simulink model "MILSIM"  (R2018b)
settings: Solver=FixedStepDiscrete  StartTime=0.0  StopTime=1000  FixedStep=0.002  RelTol=1e-3
undefined symbols (not defined in the file): alt, ax_cmd, ay_cmd, cmd_1, cmd_2, cmd_mask, command, DiscIntNeverNeededParam, FMS_Cmd, frame, lat, lon, mode, PilotMode, pitch, pitchspeed, psi_cmd, psi_rate_cmd, roll, rollspeed, serial, stick_pitch, stick_roll, stick_throttle, stick_yaw, timestamp, u_cmd, v_cmd, valid_items, VTOLMode, vx, vy, vz, x, x_cmd, xacc, y, y_cmd, yacc, yaw, yawspeed, z, z_cmd, zacc
libraries: hdlsllib x9, vrlib x2, instrumentlib x2, aerolibfltsims x2, aerolibutil x2, dspnetwork x2, simulink x1, aerolibanimutils x1
settings Model: Creator=jc  LastModifiedBy=spy
settings OptimizationCC: DefaultParameterBehavior=Inlined  DefaultUnderspecifiedDataType=single  EnhancedBackFolding=on  PassReuseOutputArgsAs=Individual arguments  OptimizeBlockOrder=speed  DifferentSizesBufferReuse=on  OptimizationCustomize=off
settings DebuggingCC: UnderspecifiedInitializationDetection=Classic  MergeDetectMultiDrivingBlocksExec=none  ParameterTunabilityLossMsg=error  UnitsInconsistencyMsg=none
settings HardwareCC: ProdBitPerPointer=32  ProdBitPerSizeT=32  ProdBitPerPtrDiffT=32  ProdLargestAtomicInteger=Long  ProdLargestAtomicFloat=Double  ProdWordSize=32  ProdHWDeviceType=ARM Compatible->ARM Cortex
settings ModelReferenceCC: UpdateModelReferenceTargets=IfOutOfDate  PropagateSignalLabelsOutOfModel=off
settings SFSimCC: MATLABDynamicMemAlloc=off
settings RTWCC: SystemTargetFile=ert.tlc  GenCodeOnly=on  TemplateMakefile=ert_default_tmf  GenerateReport=on  IncludeHyperlinkInReport=on  LaunchReport=on  GenerateTraceInfo=on  GenerateTraceReport=on  GenerateTraceReportSl=on  GenerateTraceReportSf=on  GenerateTraceReportEml=on
settings CodeAppCC: ForceParamTrailComments=on  IgnoreCustomStorageClasses=off  OperatorAnnotations=on  SimulinkDataObjDesc=on  SFDataObjDesc=on  InsertBlockDesc=on
settings ERTTargetCC: TargetLangStandard=C99 (ISO)  GenerateSampleERTMain=on  InlinedParameterPlacement=NonHierarchical  ERTCustomFileTemplate=example_file_process.tlc

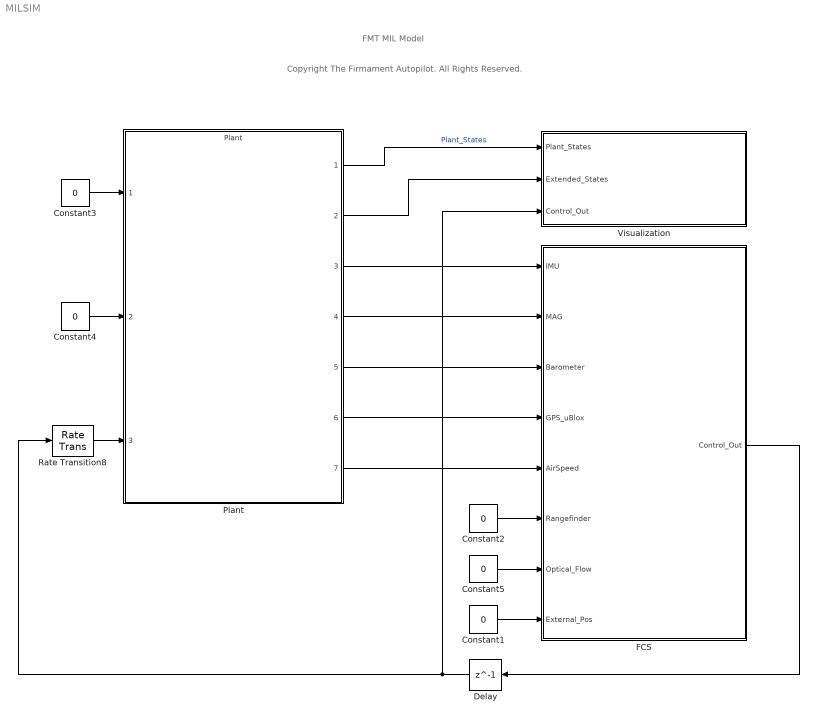
== system MILSIM ==
  note: FMT MIL Model
  note: Copyright The Firmament Autopilot. All Rights Reserved.
  Constant1 : Constant  Value=0  OutDataTypeStr=Bus: External_Pos_Bus
  Constant2 : Constant  Value=0  OutDataTypeStr=Bus: Rangefinder_Bus
  Constant3 : Constant  Value=0  OutDataTypeStr=Bus: Environment_Info_Bus
  Constant4 : Constant  Value=0  OutDataTypeStr=Bus: States_Init_Bus
  Constant5 : Constant  Value=0  OutDataTypeStr=Bus: Optical_Flow_Bus
  Delay : Delay  DelayLength=1
  FCS : Subsystem  TreatAsAtomicUnit=on
  Plant : ModelReference  ModelNameDialog=Plant.slx  ModelReferenceVersion=1.1206
  Rate Transition8 : RateTransition  OutPortSampleTime=PLANT_CONST.dt
  Visualization : Subsystem  TreatAsAtomicUnit=on
  wires:
  Plant/1 -> Visualization/1(Plant_States)  "Plant_States"
  Delay/1 -> Visualization/3(Control_Out), Rate Transition8/1
  Plant/2 -> Visualization/2(Extended_States)
  Plant/3 -> FCS/1(IMU)
  Plant/4 -> FCS/2(MAG)
  Plant/5 -> FCS/3(Barometer)
  FCS/1(Control_Out) -> Delay/1
  Constant2/1 -> FCS/6(Rangefinder)
  Constant5/1 -> FCS/7(Optical_Flow)
  Plant/7 -> FCS/5(AirSpeed)
  Constant1/1 -> FCS/8(External_Pos)
  Constant3/1 -> Plant/1
  Rate Transition8/1 -> Plant/3
  Constant4/1 -> Plant/2
  Plant/6 -> FCS/4(GPS_uBlox)

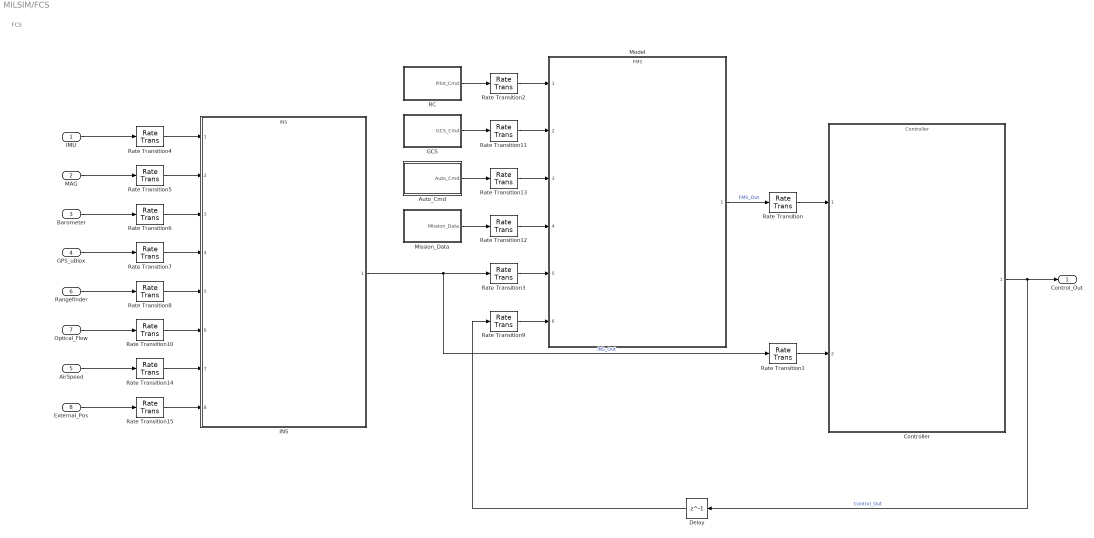
== system MILSIM/FCS ==
  note: FCS
  IMU : Inport
  MAG : Inport  Port=2
  Barometer : Inport  Port=3
  GPS_uBlox : Inport  Port=4
  AirSpeed : Inport  Port=5
  Rangefinder : Inport  Port=6
  Optical_Flow : Inport  Port=7
  External_Pos : Inport  Port=8
  Auto_Cmd : Subsystem
  Controller : ModelReference  ModelNameDialog=Controller.slx  ModelReferenceVersion=1.1001
  Delay : Delay  DelayLength=1
  GCS : Subsystem
  INS : ModelReference  ModelNameDialog=INS.slx  ModelReferenceVersion=1.4483
  Mission_Data : Subsystem
  Model : ModelReference  ModelNameDialog=FMS.slx  ModelReferenceVersion=1.2293
  RC : Subsystem  VariantControlMode=Label  Variant=on  VariantControl=Variant1  LabelModeActiveChoice=VIRTUAL_INPUT
  Rate Transition : RateTransition  OutPortSampleTime=CONTROL_CONST.dt
  Rate Transition1 : RateTransition  OutPortSampleTime=CONTROL_CONST.dt
  Rate Transition{4..8,10,14..15} (8 alike) : RateTransition  OutPortSampleTime=INS_CONST.dt
  Rate Transition{2..3,9,11..13} (6 alike) : RateTransition  OutPortSampleTime=FMS_CONST.dt
  Control_Out : Outport
  wires:
  INS/1 -> Rate Transition3/1, Rate Transition1/1  "INS_Out"
  Rate Transition2/1 -> Model/1
  Rate Transition4/1 -> INS/1
  Rate Transition/1 -> Controller/1
  Rate Transition1/1 -> Controller/2
  RC/1(" Pilot_Cmd") -> Rate Transition2/1
  Rangefinder/1 -> Rate Transition8/1
  Model/1 -> Rate Transition/1  "FMS_Out"
  Barometer/1 -> Rate Transition6/1
  Rate Transition3/1 -> Model/5
  MAG/1 -> Rate Transition5/1
  Rate Transition9/1 -> Model/6
  Controller/1 -> Delay/1, Control_Out/1  "Control_Out"
  IMU/1 -> Rate Transition4/1
  Delay/1 -> Rate Transition9/1
  Optical_Flow/1 -> Rate Transition10/1
  Rate Transition5/1 -> INS/2
  Rate Transition6/1 -> INS/3
  Rate Transition7/1 -> INS/4
  Rate Transition8/1 -> INS/5
  Rate Transition10/1 -> INS/6
  GPS_uBlox/1 -> Rate Transition7/1
  Rate Transition13/1 -> Model/3
  GCS/1(GCS_Cmd) -> Rate Transition11/1
  Rate Transition11/1 -> Model/2
  Mission_Data/1(Mission_Data) -> Rate Transition12/1
  Rate Transition12/1 -> Model/4
  Rate Transition14/1 -> INS/7
  Auto_Cmd/1(Auto_Cmd) -> Rate Transition13/1
  AirSpeed/1 -> Rate Transition14/1
  External_Pos/1 -> Rate Transition15/1
  Rate Transition15/1 -> INS/8

== system MILSIM/Visualization ==
  Plant_States : Inport
  Extended_States : Inport  Port=2
  Control_Out : Inport  Port=3
  3D_Visualization : Subsystem  VariantControlMode=Label  Variant=on  LabelModeActiveChoice=UE4
  Simulation Pace : aerolibanimutils/Simulation Pace  SimulationPace=1  SleepMode=Auto  OutputPaceError=off  SampleTime=-1
  wires:
  Plant_States/1 -> 3D_Visualization/1(Plant_States)
  Extended_States/1 -> 3D_Visualization/2(Extended_States)
  Control_Out/1 -> 3D_Visualization/3(Control_Out)

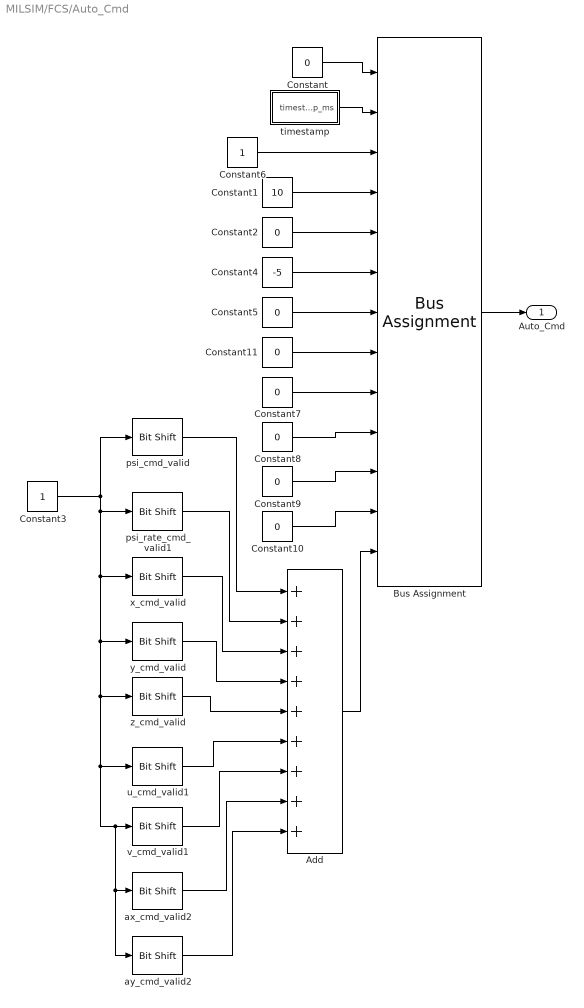
== system MILSIM/FCS/Auto_Cmd ==
  Add : Sum  Inputs=+++++++++
  Bus Assignment : BusAssignment  AssignedSignals=timestamp,frame,x_cmd,y_cmd,z_cmd,psi_cmd,psi_rate_cmd,u_cmd,v_cmd,ax_cmd,ay_cmd,cmd_mask
  Constant : Constant  Value=0  OutDataTypeStr=Bus: Auto_Cmd_Bus
  Constant1 : Constant  Value=10  OutDataTypeStr=single
  Constant{2,5,7..11} (7 alike) : Constant  Value=0  OutDataTypeStr=single
  Constant3 : Constant  OutDataTypeStr=uint32
  Constant4 : Constant  Value=-5  OutDataTypeStr=single
  Constant6 : Constant  OutDataTypeStr=uint8
  ax_cmd_valid2 : hdlsllib/Logic and Bit Operations/Bit Shift  mode=Shift Left Logical  N=16
      settings: SourceProductName=HDL Coder  SourceProductBaseCode=HD
  ay_cmd_valid2 : hdlsllib/Logic and Bit Operations/Bit Shift  mode=Shift Left Logical  N=17
      settings: SourceProductName=HDL Coder  SourceProductBaseCode=HD
  psi_cmd_valid : hdlsllib/Logic and Bit Operations/Bit Shift  mode=Shift Left Logical  N=5
      settings: SourceProductName=HDL Coder  SourceProductBaseCode=HD
  psi_rate_cmd_valid1 : hdlsllib/Logic and Bit Operations/Bit Shift  mode=Shift Left Logical  N=6
      settings: SourceProductName=HDL Coder  SourceProductBaseCode=HD
  timestamp : Subsystem  mask{sample_time=2}
      mask prompts: sample_time "sample time (ms)"
  u_cmd_valid1 : hdlsllib/Logic and Bit Operations/Bit Shift  mode=Shift Left Logical  N=13
      settings: SourceProductName=HDL Coder  SourceProductBaseCode=HD
  v_cmd_valid1 : hdlsllib/Logic and Bit Operations/Bit Shift  mode=Shift Left Logical  N=14
      settings: SourceProductName=HDL Coder  SourceProductBaseCode=HD
  x_cmd_valid : hdlsllib/Logic and Bit Operations/Bit Shift  mode=Shift Left Logical  N=7
      settings: SourceProductName=HDL Coder  SourceProductBaseCode=HD
  y_cmd_valid : hdlsllib/Logic and Bit Operations/Bit Shift  mode=Shift Left Logical  N=8
      settings: SourceProductName=HDL Coder  SourceProductBaseCode=HD
  z_cmd_valid : hdlsllib/Logic and Bit Operations/Bit Shift  mode=Shift Left Logical  N=9
      settings: SourceProductName=HDL Coder  SourceProductBaseCode=HD
  Auto_Cmd : Outport
  wires:
  timestamp/1(timestamp_ms) -> Bus Assignment/2
  Constant/1 -> Bus Assignment/1
  Bus Assignment/1 -> Auto_Cmd/1
  Constant3/1 -> psi_rate_cmd_valid1/1, ay_cmd_valid2/1, ax_cmd_valid2/1, v_cmd_valid1/1, u_cmd_valid1/1, z_cmd_valid/1, y_cmd_valid/1, x_cmd_valid/1, psi_cmd_valid/1
  Constant5/1 -> Bus Assignment/7
  Constant4/1 -> Bus Assignment/6
  Constant2/1 -> Bus Assignment/5
  Constant1/1 -> Bus Assignment/4
  Constant6/1 -> Bus Assignment/3
  Constant7/1 -> Bus Assignment/9
  Constant8/1 -> Bus Assignment/10
  Constant9/1 -> Bus Assignment/11
  Constant10/1 -> Bus Assignment/12
  Add/1 -> Bus Assignment/13
  Constant11/1 -> Bus Assignment/8
  psi_cmd_valid/1 -> Add/1
  psi_rate_cmd_valid1/1 -> Add/2
  x_cmd_valid/1 -> Add/3
  y_cmd_valid/1 -> Add/4
  z_cmd_valid/1 -> Add/5
  u_cmd_valid1/1 -> Add/6
  v_cmd_valid1/1 -> Add/7
  ax_cmd_valid2/1 -> Add/8
  ay_cmd_valid2/1 -> Add/9

== system MILSIM/FCS/GCS ==
  Bus Assignment : BusAssignment  AssignedSignals=timestamp,mode,cmd_1
  Constant : Constant  Value=0  OutDataTypeStr=Bus: GCS_Cmd_Bus
  Constant1 : Constant  Value=FMS_Cmd.None
  Constant4 : Constant  Value=PilotMode.None  SampleTime=-1
  Data Type Conversion : DataTypeConversion
  Data Type Conversion1 : DataTypeConversion
  timestamp : Subsystem  mask{sample_time=2}
      mask prompts: sample_time "sample time (ms)"
  GCS_Cmd : Outport
  wires:
  Constant1/1 -> Data Type Conversion1/1
  Bus Assignment/1 -> GCS_Cmd/1
  Data Type Conversion1/1 -> Bus Assignment/4
  Constant/1 -> Bus Assignment/1
  timestamp/1(timestamp_ms) -> Bus Assignment/2
  Constant4/1 -> Data Type Conversion/1
  Data Type Conversion/1 -> Bus Assignment/3

== system MILSIM/FCS/Mission_Data ==
  Bus Assignment : BusAssignment  AssignedSignals=timestamp,valid_items,command,x,y,z
  Constant : Constant  OutDataTypeStr=Inherit: Inherit via back propagation
  Constant1 : Constant  Value=4  OutDataTypeStr=Inherit: Inherit via back propagation
  Constant2 : Constant  Value=0  OutDataTypeStr=Bus: Mission_Data_Bus
  Constant3 : Constant  Value=[22 16 16 20 0 0 0 0]  OutDataTypeStr=Inherit: Inherit via back propagation
  Constant4 : Constant  Value=[376277883 376280341 376277815 0 0 0 0 0]  OutDataTypeStr=Inherit: Inherit via back propagation
  Constant5 : Constant  Value=[-1223895080 -1223892241 -1223890046 0 0 0 0 0]  OutDataTypeStr=Inherit: Inherit via back propagation
  Constant6 : Constant  Value=[5 10 5 0 0 0 0 0]  OutDataTypeStr=Inherit: Inherit via back propagation
  Mission_Data : Outport
  wires:
  Constant6/1 -> Bus Assignment/7
  Constant5/1 -> Bus Assignment/6
  Constant4/1 -> Bus Assignment/5
  Constant2/1 -> Bus Assignment/1
  Constant1/1 -> Bus Assignment/3
  Constant/1 -> Bus Assignment/2
  Constant3/1 -> Bus Assignment/4
  Bus Assignment/1 -> Mission_Data/1

== system MILSIM/FCS/RC ==
  Joystick : Subsystem  VariantControl=JOYSTICK_INPUT
  Mavlink : Subsystem  VariantControl=MAVLINK_INPUT
  None : Subsystem  VariantControl=NONE_INPUT
  Virtual : Subsystem  VariantControl=VIRTUAL_INPUT
  " Pilot_Cmd" : Outport

== system MILSIM/Visualization/3D_Visualization ==
  Plant_States : Inport
  Extended_States : Inport  Port=2
  Control_Out : Inport  Port=3
  Flightgear : Subsystem  VariantControl=Flightgear
  Matlab_3D : Subsystem  VariantControl=Matlab_3D
  UE4 : Subsystem  VariantControl=UE4

== system MILSIM/FCS/Auto_Cmd/timestamp ==
  Constant : Constant  Value=sample_time
  Data Type Conversion : DataTypeConversion  OutDataTypeStr=uint32
  Discrete-Time Integrator : DiscreteIntegrator  IntegratorMethod=Accumulation: Forward Euler  SampleTime=-1  ICPrevOutput=DiscIntNeverNeededParam  ICPrevScaledInput=DiscIntNeverNeededParam
  timestamp_ms : Outport
  wires:
  Data Type Conversion/1 -> timestamp_ms/1
  Constant/1 -> Discrete-Time Integrator/1
  Discrete-Time Integrator/1 -> Data Type Conversion/1

== system MILSIM/FCS/GCS/timestamp ==
  Constant : Constant  Value=sample_time
  Data Type Conversion : DataTypeConversion  OutDataTypeStr=uint32
  Discrete-Time Integrator : DiscreteIntegrator  IntegratorMethod=Accumulation: Forward Euler  SampleTime=-1  ICPrevOutput=DiscIntNeverNeededParam  ICPrevScaledInput=DiscIntNeverNeededParam
  timestamp_ms : Outport
  wires:
  Discrete-Time Integrator/1 -> Data Type Conversion/1
  Constant/1 -> Discrete-Time Integrator/1
  Data Type Conversion/1 -> timestamp_ms/1

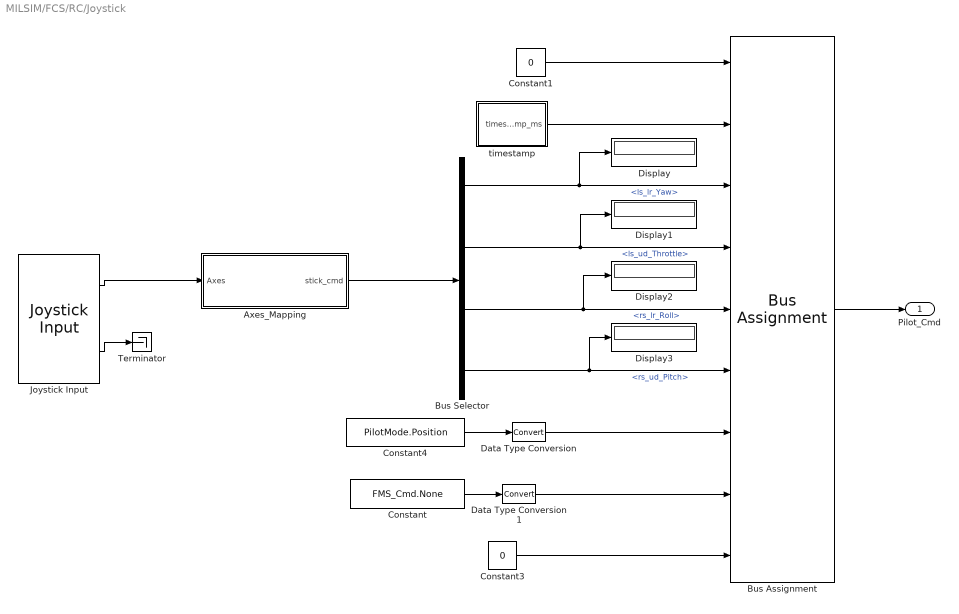
== system MILSIM/FCS/RC/Joystick ==
  Axes_Mapping : Subsystem
  Bus Assignment : BusAssignment  AssignedSignals=timestamp,stick_yaw,stick_throttle,stick_roll,stick_pitch,mode,cmd_1,cmd_2
  Bus Selector : BusSelector  OutputSignals=ls_lr_Yaw,ls_ud_Throttle,rs_lr_Roll,rs_ud_Pitch
  Constant : Constant  Value=FMS_Cmd.None
  Constant1 : Constant  Value=0  OutDataTypeStr=Bus: Pilot_Cmd_Bus
  Constant3 : Constant  Value=0  OutDataTypeStr=Inherit: Inherit via back propagation
  Constant4 : Constant  Value=PilotMode.Position  SampleTime=-1
  Data Type Conversion : DataTypeConversion
  Data Type Conversion1 : DataTypeConversion
  Display{,1..3} (4 alike) : Display
  Joystick Input : vrlib/Joystick Input  joyid=1  adjustports=off  forcefeed=off
      settings: SourceProductBaseCode=VR
  Terminator : Terminator
  timestamp : Subsystem  mask{sample_time=2}
      mask prompts: sample_time "sample time (ms)"
  Pilot_Cmd : Outport  OutDataTypeStr=Bus: Pilot_Cmd_Bus
  wires:
  Constant1/1 -> Bus Assignment/1
  Data Type Conversion1/1 -> Bus Assignment/8
  timestamp/1(timestamp_ms) -> Bus Assignment/2
  Bus Selector/2 -> Display1/1, Bus Assignment/4  "<ls_ud_Throttle>"
  Bus Selector/3 -> Display2/1, Bus Assignment/5  "<rs_lr_Roll>"
  Axes_Mapping/1(stick_cmd) -> Bus Selector/1
  Bus Selector/1 -> Display/1, Bus Assignment/3  "<ls_lr_Yaw>"
  Constant3/1 -> Bus Assignment/9
  Bus Assignment/1 -> Pilot_Cmd/1
  Bus Selector/4 -> Display3/1, Bus Assignment/6  "<rs_ud_Pitch>"
  Constant4/1 -> Data Type Conversion/1
  Joystick Input/1 -> Axes_Mapping/1(Axes)
  Joystick Input/2 -> Terminator/1
  Data Type Conversion/1 -> Bus Assignment/7
  Constant/1 -> Data Type Conversion1/1

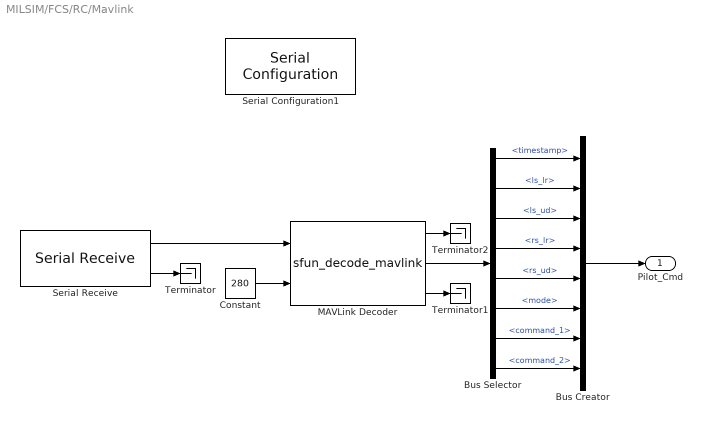
== system MILSIM/FCS/RC/Mavlink ==
  Bus Creator : BusCreator  Inputs=8
  Bus Selector : BusSelector  OutputSignals=timestamp,ls_lr,ls_ud,rs_lr,rs_ud,mode,command_1,command_2
  Constant : Constant  Value=280  OutDataTypeStr=uint16
  MAVLink Decoder : S-Function  FunctionName=sfun_decode_mavlink  SFunctionDeploymentMode=off  EnableBusSupport=off
  Serial Configuration1 : instrumentlib/Serial Configuration  Priority=-200000  ComPortMenu=<Please select a port...>  ComPort=COM9  ObjConstructor=serial('COM9');  BaudRate=9600  DataBits=8  Parity=none  StopBits=1  FlowControl=none  Timeout=10  ByteOrder=LittleEndian
  Serial Receive : instrumentlib/Serial Receive  ComPortMenu=<Please select a port...>  ComPort=COM9  ObjConstructor=serial('COM9');  Terminator=<none>  DataSize=280  DataType=uint8  EnableBlockingMode=off  ActionDataUnavailable=Output last received value  CustomValue=0  SampleTime=-1
  Terminator : Terminator
  Terminator1 : Terminator
  Terminator2 : Terminator
  Pilot_Cmd : Outport
  wires:
  Serial Receive/1 -> MAVLink Decoder/1
  Serial Receive/2 -> Terminator/1
  Bus Selector/1 -> Bus Creator/1  "<timestamp>"
  Bus Selector/2 -> Bus Creator/2  "<ls_lr>"
  Bus Selector/3 -> Bus Creator/3  "<ls_ud>"
  Bus Selector/4 -> Bus Creator/4  "<rs_lr>"
  Bus Selector/5 -> Bus Creator/5  "<rs_ud>"
  Bus Selector/6 -> Bus Creator/6  "<mode>"
  Bus Selector/7 -> Bus Creator/7  "<command_1>"
  Bus Selector/8 -> Bus Creator/8  "<command_2>"
  Bus Creator/1 -> Pilot_Cmd/1
  MAVLink Decoder/2 -> Bus Selector/1
  Constant/1 -> MAVLink Decoder/2
  MAVLink Decoder/3 -> Terminator1/1
  MAVLink Decoder/1 -> Terminator2/1

== system MILSIM/FCS/RC/None ==
  Constant : Constant  Value=0  OutDataTypeStr=Bus: Pilot_Cmd_Bus
  Pilot_Cmd : Outport  OutDataTypeStr=Bus: Pilot_Cmd_Bus
  wires:
  Constant/1 -> Pilot_Cmd/1

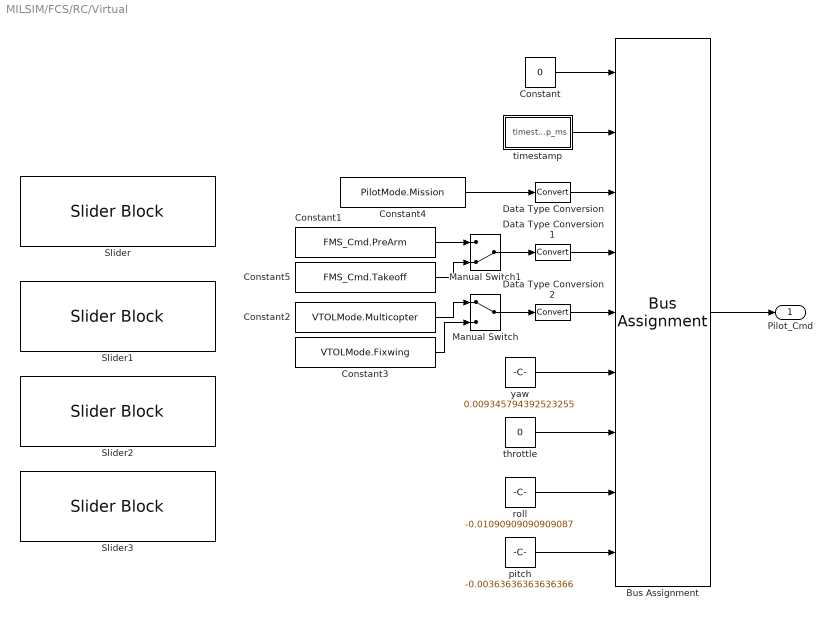
== system MILSIM/FCS/RC/Virtual ==
  Bus Assignment : BusAssignment  AssignedSignals=timestamp,mode,cmd_1,cmd_2,stick_yaw,stick_throttle,stick_roll,stick_pitch
  Constant : Constant  Value=0  OutDataTypeStr=Bus: Pilot_Cmd_Bus
  Constant1 : Constant  Value=FMS_Cmd.PreArm
  Constant2 : Constant  Value=VTOLMode.Multicopter
  Constant3 : Constant  Value=VTOLMode.Fixwing
  Constant4 : Constant  Value=PilotMode.Mission  SampleTime=-1
  Constant5 : Constant  Value=FMS_Cmd.Takeoff
  Data Type Conversion : DataTypeConversion
  Data Type Conversion1 : DataTypeConversion
  Data Type Conversion2 : DataTypeConversion
  Manual Switch : ManualSwitch
  Manual Switch1 : ManualSwitch  CurrentSetting=0
  Slider : SliderBlock  WebBlockId=1308  ScaleMin=-1  ScaleMax=1
  Slider1 : SliderBlock  WebBlockId=1315  ScaleMin=-1  ScaleMax=1
  Slider2 : SliderBlock  WebBlockId=1316  ScaleMin=-1  ScaleMax=1
  Slider3 : SliderBlock  WebBlockId=1317  ScaleMin=-1  ScaleMax=1
  pitch : Constant  Value=-0.00363636363636366  OutDataTypeStr=single
  roll : Constant  Value=-0.01090909090909087  OutDataTypeStr=single
  throttle : Constant  Value=0  OutDataTypeStr=single
  timestamp : Subsystem  mask{sample_time=2}
      mask prompts: sample_time "sample time (ms)"
  yaw : Constant  Value=0.009345794392523255  OutDataTypeStr=single
  Pilot_Cmd : Outport  OutDataTypeStr=Bus: Pilot_Cmd_Bus
  wires:
  Bus Assignment/1 -> Pilot_Cmd/1
  Constant/1 -> Bus Assignment/1
  timestamp/1(timestamp_ms) -> Bus Assignment/2
  Constant4/1 -> Data Type Conversion/1
  Data Type Conversion/1 -> Bus Assignment/3
  Data Type Conversion1/1 -> Bus Assignment/4
  pitch/1 -> Bus Assignment/9
  roll/1 -> Bus Assignment/8
  throttle/1 -> Bus Assignment/7
  yaw/1 -> Bus Assignment/6
  Constant2/1 -> Manual Switch/1
  Constant3/1 -> Manual Switch/2
  Manual Switch/1 -> Data Type Conversion2/1
  Data Type Conversion2/1 -> Bus Assignment/5
  Manual Switch1/1 -> Data Type Conversion1/1
  Constant1/1 -> Manual Switch1/1
  Constant5/1 -> Manual Switch1/2

== system MILSIM/Visualization/3D_Visualization/Flightgear ==
  Plant_States : Inport
  Extended_States : Inport  Port=2
  Bus Selector : BusSelector  OutputSignals=phi,theta,psi,lon,lat,alt
  Bus Selector2 : BusSelector  OutputSignals=prop_vel
  Mux : Mux  Inputs=3
  Mux1 : Mux  Inputs=3
  Selector1 : Selector  InputPortWidth=8  IndexOptions=Index vector (dialog)  Indices=[1:4]  OutputSizes=1
  Virtualization : Subsystem
  wires:
  Selector1/1 -> Virtualization/3(Prop_Rot_radPs)
  Mux/1 -> Virtualization/1(Euler)
  Mux1/1 -> Virtualization/2(Pos)
  Bus Selector2/1 -> Selector1/1  "<prop_vel>"
  Bus Selector/5 -> Mux1/2  "<lat>"
  Extended_States/1 -> Bus Selector2/1
  Plant_States/1 -> Bus Selector/1
  Bus Selector/2 -> Mux/2  "<theta>"
  Bus Selector/1 -> Mux/1  "<phi>"
  Bus Selector/6 -> Mux1/3  "<alt>"
  Bus Selector/4 -> Mux1/1  "<lon>"
  Bus Selector/3 -> Mux/3  "<psi>"

== system MILSIM/Visualization/3D_Visualization/Matlab_3D ==
  Plant_States : Inport
  Extended_States : Inport  Port=2
  Bus Selector : BusSelector  OutputSignals=phi,theta,psi,x_R,y_R,h_R
  Bus Selector2 : BusSelector  OutputSignals=prop_vel
  Gain : Gain  Gain=-1
  Mux : Mux  Inputs=3
  Mux1 : Mux  Inputs=3
  Selector1 : Selector  InputPortWidth=8  IndexOptions=Index vector (dialog)  Indices=[1:4]  OutputSizes=1
  Visualization : Subsystem
  wires:
  Bus Selector/6 -> Gain/1  "<h_R>"
  Bus Selector/3 -> Mux/3  "<psi>"
  Bus Selector/4 -> Mux1/1  "<x_R>"
  Bus Selector2/1 -> Selector1/1  "<prop_vel>"
  Bus Selector/5 -> Mux1/2  "<y_R>"
  Bus Selector/1 -> Mux/1  "<phi>"
  Selector1/1 -> Visualization/3(Prop_Rot_radPs)
  Bus Selector/2 -> Mux/2  "<theta>"
  Mux/1 -> Visualization/1(Euler)
  Mux1/1 -> Visualization/2(Pos)
  Extended_States/1 -> Bus Selector2/1
  Plant_States/1 -> Bus Selector/1
  Gain/1 -> Mux1/3

== system MILSIM/Visualization/3D_Visualization/UE4 ==
  Plant_States : Inport
  Extended_States : Inport  Port=2
  Control_Out : Inport  Port=3
  Bus Selector : BusSelector  OutputSignals=timestamp
  Detect Change : simulink/Logic and Bit Operations/Detect Change  vinit=0  OutDataTypeStr=boolean
  Pulse Generator : DiscretePulseGenerator  Period=5  SampleTime=0.002
  Send_Hil_Actuator_Controls : Subsystem
  Send_Hil_State : Subsystem
  Terminator : Terminator
  wires:
  Extended_States/1 -> Terminator/1
  Plant_States/1 -> Send_Hil_State/1(Plant_States)
  Control_Out/1 -> Bus Selector/1, Send_Hil_Actuator_Controls/1(Control_Out)
  Bus Selector/1 -> Detect Change/1  "<timestamp>"
  Detect Change/1 -> Send_Hil_Actuator_Controls/Enable
  Pulse Generator/1 -> Send_Hil_State/Enable

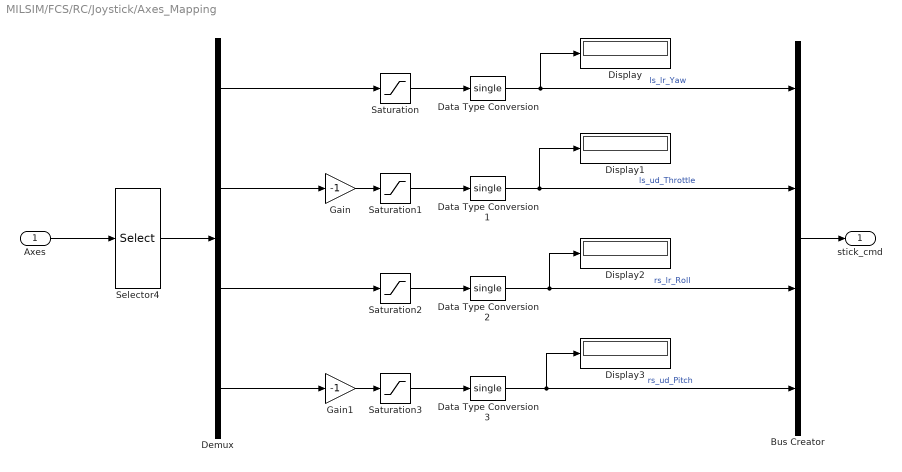
== system MILSIM/FCS/RC/Joystick/Axes_Mapping ==
  Axes : Inport
  Bus Creator : BusCreator  Inputs=4
  Data Type Conversion{,1..3} (4 alike) : DataTypeConversion  OutDataTypeStr=single
  Demux : Demux
  Display{,1..3} (4 alike) : Display
  Gain : Gain  Gain=-1  OutDataTypeStr=Inherit: Same as input
  Gain1 : Gain  Gain=-1  OutDataTypeStr=Inherit: Same as input
  Saturation{,1..3} (4 alike) : Saturate  UpperLimit=1  LowerLimit=-1
  Selector4 : Selector  InputPortWidth=8  IndexOptions=Index vector (dialog)  Indices=[1 2 4 5]  OutputSizes=1
  stick_cmd : Outport
  wires:
  Data Type Conversion1/1 -> Display1/1, Bus Creator/2  "ls_ud_Throttle"
  Data Type Conversion2/1 -> Display2/1, Bus Creator/3  "rs_lr_Roll"
  Gain/1 -> Saturation1/1
  Gain1/1 -> Saturation3/1
  Data Type Conversion3/1 -> Display3/1, Bus Creator/4  "rs_ud_Pitch"
  Data Type Conversion/1 -> Display/1, Bus Creator/1  "ls_lr_Yaw"
  Bus Creator/1 -> stick_cmd/1
  Saturation/1 -> Data Type Conversion/1
  Saturation1/1 -> Data Type Conversion1/1
  Saturation2/1 -> Data Type Conversion2/1
  Saturation3/1 -> Data Type Conversion3/1
  Demux/1 -> Saturation/1
  Demux/2 -> Gain/1
  Demux/3 -> Saturation2/1
  Demux/4 -> Gain1/1
  Axes/1 -> Selector4/1
  Selector4/1 -> Demux/1

== system MILSIM/FCS/RC/Joystick/timestamp ==
  Constant : Constant  Value=sample_time
  Data Type Conversion : DataTypeConversion  OutDataTypeStr=uint32
  Discrete-Time Integrator : DiscreteIntegrator  IntegratorMethod=Accumulation: Forward Euler  SampleTime=-1  ICPrevOutput=DiscIntNeverNeededParam  ICPrevScaledInput=DiscIntNeverNeededParam
  timestamp_ms : Outport
  wires:
  Discrete-Time Integrator/1 -> Data Type Conversion/1
  Constant/1 -> Discrete-Time Integrator/1
  Data Type Conversion/1 -> timestamp_ms/1

== system MILSIM/FCS/RC/Virtual/timestamp ==
  Constant : Constant  Value=sample_time
  Data Type Conversion : DataTypeConversion  OutDataTypeStr=uint32
  Discrete-Time Integrator : DiscreteIntegrator  IntegratorMethod=Accumulation: Forward Euler  SampleTime=-1  ICPrevOutput=DiscIntNeverNeededParam  ICPrevScaledInput=DiscIntNeverNeededParam
  timestamp_ms : Outport
  wires:
  Discrete-Time Integrator/1 -> Data Type Conversion/1
  Constant/1 -> Discrete-Time Integrator/1
  Data Type Conversion/1 -> timestamp_ms/1

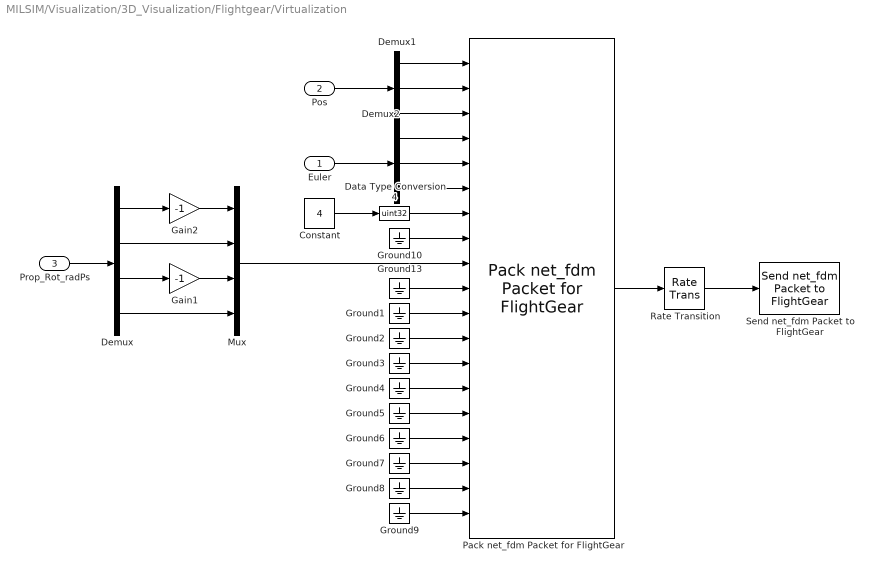
== system MILSIM/Visualization/3D_Visualization/Flightgear/Virtualization ==
  Euler : Inport
  Pos : Inport  Port=2
  Prop_Rot_radPs : Inport  Port=3
  Constant : Constant  Value=4
  Data Type Conversion4 : DataTypeConversion  OutDataTypeStr=uint32
  Demux : Demux
  Demux1 : Demux  Outputs=3
  Demux2 : Demux  Outputs=3
  Gain1 : Gain  Gain=-1  OutDataTypeStr=Inherit: Same as input
  Gain2 : Gain  Gain=-1  OutDataTypeStr=Inherit: Same as input
  Ground{1..10,13} (11 alike) : Ground
  Mux : Mux
  Pack net_fdm Packet for FlightGear : aerolibfltsims/Pack net_fdm Packet for FlightGear  FlightGearVersion=v2016.1  ShowPositionAttitudeInputs=on  ShowVelocityAccelerationInputs=off  ShowControlSurfacePositionInputs=off  ShowEngineFuelInputs=on  ShowLandingGearInputs=off  ShowEnvironmentInputs=off  SampleTime=1/50  packetVersion=24
      settings: SourceProductName=Aerospace Blockset  SourceProductBaseCode=AE
  Rate Transition : RateTransition
  Send net_fdm Packet to FlightGear : aerolibfltsims/Send net_fdm Packet to FlightGear  DestinationIpAddress=127.0.0.1  DestinationPort=5502  LocalIpPort=-1  varLen=off  SampleTime=1/25
      settings: SourceProductName=Aerospace Blockset  SourceProductBaseCode=AE
  wires:
  Euler/1 -> Demux2/1
  Demux/4 -> Mux/4
  Pos/1 -> Demux1/1
  Prop_Rot_radPs/1 -> Demux/1
  Demux1/1 -> Pack net_fdm Packet for FlightGear/1
  Rate Transition/1 -> Send net_fdm Packet to FlightGear/1
  Demux2/1 -> Pack net_fdm Packet for FlightGear/4
  Demux2/3 -> Pack net_fdm Packet for FlightGear/6
  Demux2/2 -> Pack net_fdm Packet for FlightGear/5
  Demux1/3 -> Pack net_fdm Packet for FlightGear/3
  Demux1/2 -> Pack net_fdm Packet for FlightGear/2
  Ground13/1 -> Pack net_fdm Packet for FlightGear/10
  Ground1/1 -> Pack net_fdm Packet for FlightGear/11
  Ground2/1 -> Pack net_fdm Packet for FlightGear/12
  Ground3/1 -> Pack net_fdm Packet for FlightGear/13
  Ground4/1 -> Pack net_fdm Packet for FlightGear/14
  Ground5/1 -> Pack net_fdm Packet for FlightGear/15
  Ground6/1 -> Pack net_fdm Packet for FlightGear/16
  Ground7/1 -> Pack net_fdm Packet for FlightGear/17
  Ground8/1 -> Pack net_fdm Packet for FlightGear/18
  Ground9/1 -> Pack net_fdm Packet for FlightGear/19
  Constant/1 -> Data Type Conversion4/1
  Data Type Conversion4/1 -> Pack net_fdm Packet for FlightGear/7
  Ground10/1 -> Pack net_fdm Packet for FlightGear/8
  Pack net_fdm Packet for FlightGear/1 -> Rate Transition/1
  Gain2/1 -> Mux/1
  Demux/1 -> Gain2/1
  Demux/2 -> Mux/2
  Demux/3 -> Gain1/1
  Mux/1 -> Pack net_fdm Packet for FlightGear/9
  Gain1/1 -> Mux/3

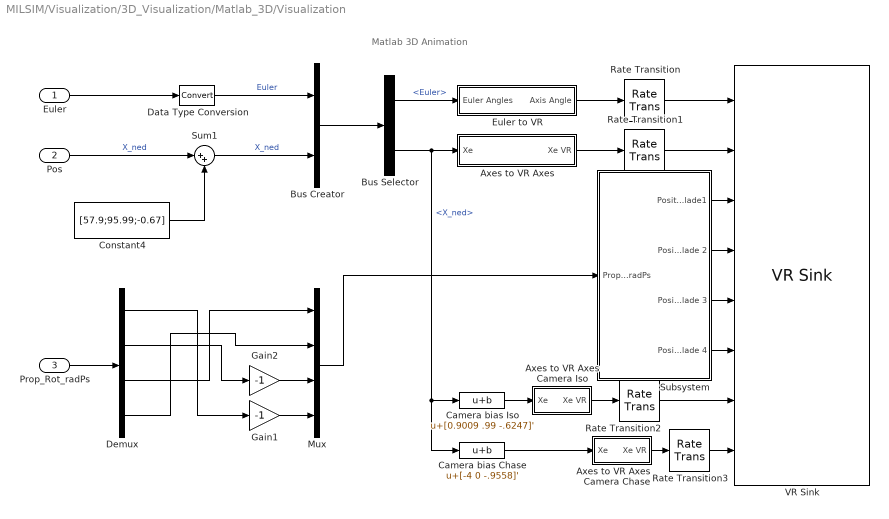
== system MILSIM/Visualization/3D_Visualization/Matlab_3D/Visualization ==
  note: Matlab 3D Animation
  Euler : Inport
  Pos : Inport  Port=2
  Prop_Rot_radPs : Inport  Port=3
  Axes to VR Axes : Subsystem
  Axes to VR Axes Camera Chase : Subsystem
  Axes to VR Axes Camera Iso : Subsystem
  Bus Creator : BusCreator  Inputs=2
  Bus Selector : BusSelector  OutputSignals=Euler,X_ned
  Camera bias Chase : Bias  Bias=[-4 0 -.9558]'
  Camera bias Iso : Bias  Bias=[0.9009 .99 -.6247]'
  Constant4 : Constant  Value=[57.9;95.99;-0.67]  OutDataTypeStr=Inherit: Inherit via back propagation
  Data Type Conversion : DataTypeConversion
  Demux : Demux
  Euler to VR : Subsystem
  Gain1 : Gain  Gain=-1  OutDataTypeStr=Inherit: Same as input
  Gain2 : Gain  Gain=-1  OutDataTypeStr=Inherit: Same as input
  Mux : Mux
  Rate Transition{,1..3} (4 alike) : RateTransition
  Subsystem : Subsystem
  Sum1 : Sum  Inputs=|++
  VR Sink : vrlib/VR Sink  InstantiateOnLoad=on  SampleTime=0.1  ViewEnable=on  RemoteChange=off  RemoteView=off  FieldsWritten=QuadBody.rotation.4.1.1.double#QuadBody.translation.3.1.1.double#Blade1.rotation.4.1.1.double#Blade3.rotation.4.1.1.double#Blade2.rotation.4.1.1.double#Blade4.rotation.4.1.1.double#IsoNoRotation.position.3.1.1.double#OnQuadNoRotation.position.3.1.1.double  WorldFileName=asbQuadcopterWorld.wrl  AutoView=off  VideoDimensions=[]  AllowVariableSize=off
      settings: SourceProductBaseCode=VR
  wires:
  Euler/1 -> Data Type Conversion/1
  Sum1/1 -> Bus Creator/2  "X_ned"
  Demux/1 -> Gain1/1
  Gain1/1 -> Mux/4
  Demux/2 -> Gain2/1
  Demux/3 -> Mux/1
  Demux/4 -> Mux/2
  Gain2/1 -> Mux/3
  Constant4/1 -> Sum1/2
  Pos/1 -> Sum1/1  "X_ned"
  Data Type Conversion/1 -> Bus Creator/1  "Euler"
  Prop_Rot_radPs/1 -> Demux/1
  Camera bias Chase/1 -> Axes to VR Axes Camera Chase/1(Xe)
  Rate Transition2/1 -> VR Sink/7
  Rate Transition3/1 -> VR Sink/8
  Euler to VR/1(Axis Angle) -> Rate Transition/1
  Subsystem/1(Position Blade1) -> VR Sink/3
  Mux/1 -> Subsystem/1(Prop_Rot_radPs)
  Subsystem/2(Position Blade 2) -> VR Sink/4
  Axes to VR Axes Camera Chase/1(Xe VR) -> Rate Transition3/1
  Bus Selector/2 -> Camera bias Chase/1, Camera bias Iso/1, Axes to VR Axes/1(Xe)  "<X_ned>"
  Axes to VR Axes Camera Iso/1(Xe VR) -> Rate Transition2/1
  Rate Transition1/1 -> VR Sink/2
  Axes to VR Axes/1(Xe VR) -> Rate Transition1/1
  Camera bias Iso/1 -> Axes to VR Axes Camera Iso/1(Xe)
  Bus Selector/1 -> Euler to VR/1(Euler Angles)  "<Euler>"
  Subsystem/4(Position Blade 4) -> VR Sink/6
  Bus Creator/1 -> Bus Selector/1
  Subsystem/3(Position Blade 3) -> VR Sink/5
  Rate Transition/1 -> VR Sink/1

== system MILSIM/Visualization/3D_Visualization/UE4/Send_Hil_Actuator_Controls ==
  Control_Out : Inport
  Enable : EnablePort
  Bias : Bias  Bias=-3
  Bus Assignment1 : BusAssignment  AssignedSignals=controls
  Bus Selector1 : BusSelector  OutputSignals=actuator_cmd
  Constant1 : Constant  Value=0  OutDataTypeStr=Bus: mavlink_hil_actuator_controls_t
  Encoder : S-Function  FunctionName=sfun_encode_msg_hil_actuator_controls  SFunctionDeploymentMode=off  EnableBusSupport=off
  Gain9 : Gain  Gain=0.02  OutDataTypeStr=single
  UDP Send2 : dspnetwork/UDP Send  remoteURL='127.0.0.1'  remotePort=14553  localURL='0.0.0.0'  localPortSource=Specify via dialog  localPort=14552  sampletime=-1  blockPlatform=HOST  separateLengthPort=0
      settings: SourceProductName=DSP System Toolbox  SourceProductBaseCode=DS
  wires:
  Bus Assignment1/1 -> Encoder/1
  Bus Selector1/1 -> Gain9/1  "<actuator_cmd>"
  Constant1/1 -> Bus Assignment1/1
  Control_Out/1 -> Bus Selector1/1
  Bias/1 -> Bus Assignment1/2
  Encoder/1 -> UDP Send2/1
  Gain9/1 -> Bias/1

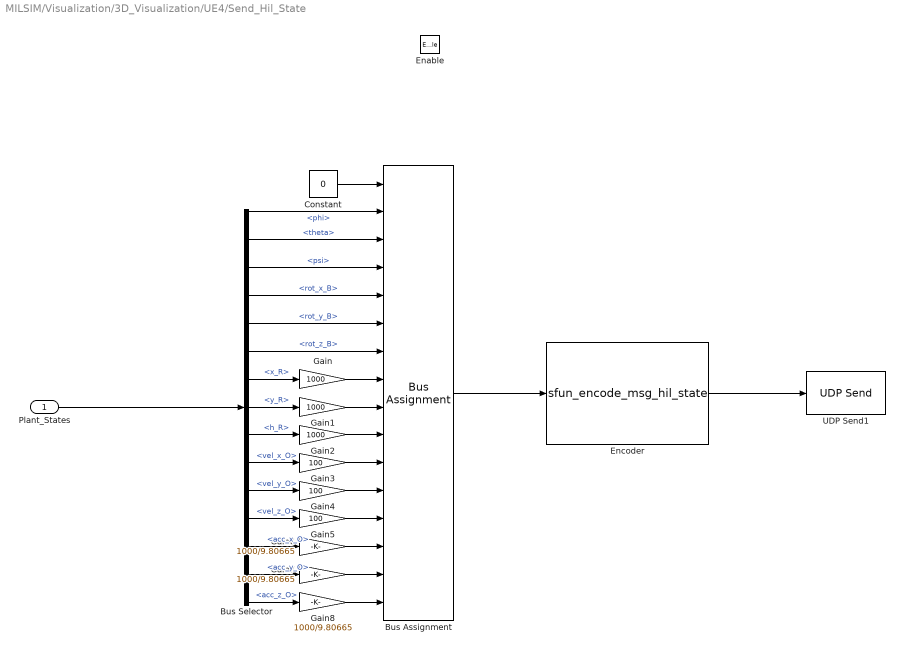
== system MILSIM/Visualization/3D_Visualization/UE4/Send_Hil_State ==
  Plant_States : Inport
  Enable : EnablePort
  Bus Assignment : BusAssignment  AssignedSignals=roll,pitch,yaw,rollspeed,yawspeed,pitchspeed,lat,lon,alt,vx,vy,vz,xacc,yacc,zacc
  Bus Selector : BusSelector  OutputSignals=phi,theta,psi,rot_x_B,rot_y_B,rot_z_B,x_R,y_R,h_R,vel_x_O,vel_y_O,vel_z_O,acc_x_O,acc_y_O,acc_z_O
  Constant : Constant  Value=0  OutDataTypeStr=Bus: mavlink_hil_state_t
  Encoder : S-Function  FunctionName=sfun_encode_msg_hil_state  SFunctionDeploymentMode=off  EnableBusSupport=off
  Gain : Gain  Gain=1000  OutDataTypeStr=int32
  Gain1 : Gain  Gain=1000  OutDataTypeStr=int32
  Gain2 : Gain  Gain=1000  OutDataTypeStr=int32
  Gain3 : Gain  Gain=100  OutDataTypeStr=int16
  Gain4 : Gain  Gain=100  OutDataTypeStr=int16
  Gain5 : Gain  Gain=100  OutDataTypeStr=int16
  Gain6 : Gain  Gain=1000/9.80665  OutDataTypeStr=int16
  Gain7 : Gain  Gain=1000/9.80665  OutDataTypeStr=int16
  Gain8 : Gain  Gain=1000/9.80665  OutDataTypeStr=int16
  UDP Send1 : dspnetwork/UDP Send  remoteURL='127.0.0.1'  remotePort=14553  localURL='0.0.0.0'  localPortSource=Specify via dialog  localPort=14552  sampletime=-1  blockPlatform=HOST  separateLengthPort=0
      settings: SourceProductName=DSP System Toolbox  SourceProductBaseCode=DS
  wires:
  Bus Selector/8 -> Gain1/1  "<y_R>"
  Constant/1 -> Bus Assignment/1
  Bus Selector/3 -> Bus Assignment/4  "<psi>"
  Bus Selector/2 -> Bus Assignment/3  "<theta>"
  Encoder/1 -> UDP Send1/1
  Bus Selector/1 -> Bus Assignment/2  "<phi>"
  Bus Selector/6 -> Bus Assignment/7  "<rot_z_B>"
  Bus Selector/7 -> Gain/1  "<x_R>"
  Gain/1 -> Bus Assignment/8
  Bus Selector/11 -> Gain4/1  "<vel_y_O>"
  Bus Selector/12 -> Gain5/1  "<vel_z_O>"
  Bus Selector/4 -> Bus Assignment/5  "<rot_x_B>"
  Gain1/1 -> Bus Assignment/9
  Bus Selector/5 -> Bus Assignment/6  "<rot_y_B>"
  Gain6/1 -> Bus Assignment/14
  Bus Selector/9 -> Gain2/1  "<h_R>"
  Gain3/1 -> Bus Assignment/11
  Gain5/1 -> Bus Assignment/13
  Bus Selector/10 -> Gain3/1  "<vel_x_O>"
  Gain8/1 -> Bus Assignment/16
  Bus Selector/14 -> Gain7/1  "<acc_y_O>"
  Bus Assignment/1 -> Encoder/1
  Gain2/1 -> Bus Assignment/10
  Gain7/1 -> Bus Assignment/15
  Gain4/1 -> Bus Assignment/12
  Plant_States/1 -> Bus Selector/1
  Bus Selector/13 -> Gain6/1  "<acc_x_O>"
  Bus Selector/15 -> Gain8/1  "<acc_z_O>"

== system MILSIM/Visualization/3D_Visualization/Matlab_3D/Visualization/Axes to VR Axes ==
  Xe : Inport
  Demux : Demux  Outputs=3
  Mux : Mux  Inputs=3
  rad-->deg1 : Gain  Gain=-1  SaturateOnIntegerOverflow=on  OutDataTypeStr=Inherit: Same as input  ParamDataTypeStr=Inherit: Same as input
  Xe VR : Outport
  wires:
  Xe/1 -> Demux/1
  Demux/1 -> Mux/1
  Demux/3 -> rad-->deg1/1
  Mux/1 -> Xe VR/1
  rad-->deg1/1 -> Mux/2
  Demux/2 -> Mux/3

== system MILSIM/Visualization/3D_Visualization/Matlab_3D/Visualization/Axes to VR Axes Camera Chase ==
  Xe : Inport
  Demux : Demux  Outputs=3
  Mux : Mux  Inputs=3
  rad-->deg1 : Gain  Gain=-1  SaturateOnIntegerOverflow=on  OutDataTypeStr=Inherit: Same as input  ParamDataTypeStr=Inherit: Same as input
  Xe VR : Outport
  wires:
  Xe/1 -> Demux/1
  Demux/1 -> Mux/1
  Demux/3 -> rad-->deg1/1
  Mux/1 -> Xe VR/1
  rad-->deg1/1 -> Mux/2
  Demux/2 -> Mux/3

== system MILSIM/Visualization/3D_Visualization/Matlab_3D/Visualization/Axes to VR Axes Camera Iso ==
  Xe : Inport
  Demux : Demux  Outputs=3
  Mux : Mux  Inputs=3
  rad-->deg1 : Gain  Gain=-1  SaturateOnIntegerOverflow=on  OutDataTypeStr=Inherit: Same as input  ParamDataTypeStr=Inherit: Same as input
  Xe VR : Outport
  wires:
  Demux/2 -> Mux/3
  rad-->deg1/1 -> Mux/2
  Mux/1 -> Xe VR/1
  Demux/3 -> rad-->deg1/1
  Demux/1 -> Mux/1
  Xe/1 -> Demux/1

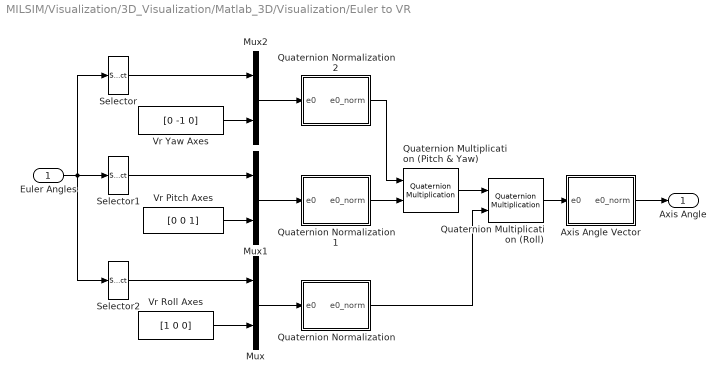
== system MILSIM/Visualization/3D_Visualization/Matlab_3D/Visualization/Euler to VR ==
  Euler Angles : Inport
  Axis Angle Vector : Subsystem
  Mux : Mux  Inputs=2
  Mux1 : Mux  Inputs=2
  Mux2 : Mux  Inputs=2
  Quaternion Multiplication (Pitch & Yaw) : aerolibutil/Quaternion Multiplication
  Quaternion Multiplication (Roll) : aerolibutil/Quaternion Multiplication
  Quaternion Normalization : Subsystem
  Quaternion Normalization1 : Subsystem
  Quaternion Normalization2 : Subsystem
  Selector : Selector  InputPortWidth=3  IndexOptions=Index vector (dialog)  Indices=[3]  OutputSizes=1
  Selector1 : Selector  InputPortWidth=3  IndexOptions=Index vector (dialog)  Indices=[2]  OutputSizes=1
  Selector2 : Selector  InputPortWidth=3  IndexOptions=Index vector (dialog)  Indices=[1]  OutputSizes=1
  Vr Pitch Axes : Constant  Value=[0 0 1]
  Vr Roll Axes : Constant  Value=[1 0 0]
  Vr Yaw Axes : Constant  Value=[0 -1 0]
  Axis Angle : Outport
  wires:
  Quaternion Multiplication (Roll)/1 -> Axis Angle Vector/1(e0)
  Axis Angle Vector/1(e0_norm) -> Axis Angle/1
  Quaternion Normalization/1(e0_norm) -> Quaternion Multiplication (Roll)/2
  Quaternion Normalization2/1(e0_norm) -> Quaternion Multiplication (Pitch & Yaw)/1
  Quaternion Normalization1/1(e0_norm) -> Quaternion Multiplication (Pitch & Yaw)/2
  Mux2/1 -> Quaternion Normalization2/1(e0)
  Mux1/1 -> Quaternion Normalization1/1(e0)
  Mux/1 -> Quaternion Normalization/1(e0)
  Selector/1 -> Mux2/1
  Vr Yaw Axes/1 -> Mux2/2
  Selector1/1 -> Mux1/1
  Vr Pitch Axes/1 -> Mux1/2
  Selector2/1 -> Mux/1
  Vr Roll Axes/1 -> Mux/2
  Euler Angles/1 -> Selector2/1, Selector1/1, Selector/1
  Quaternion Multiplication (Pitch & Yaw)/1 -> Quaternion Multiplication (Roll)/1

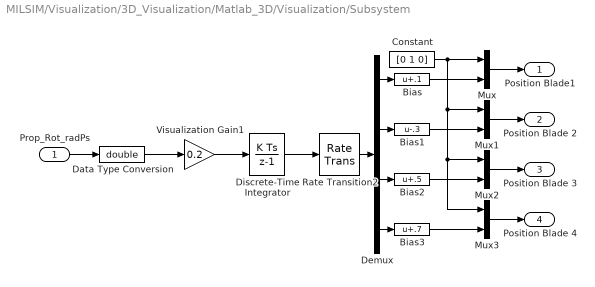
== system MILSIM/Visualization/3D_Visualization/Matlab_3D/Visualization/Subsystem ==
  Prop_Rot_radPs : Inport
  Bias : Bias  Bias=.1
  Bias1 : Bias  Bias=-.3
  Bias2 : Bias  Bias=.5
  Bias3 : Bias  Bias=.7
  Constant : Constant  Value=[0 1 0]
  Data Type Conversion : DataTypeConversion  OutDataTypeStr=double
  Demux : Demux
  Discrete-Time Integrator : DiscreteIntegrator  InitialCondition="[.1  .2 -.3 -.4]"  SampleTime=-1  UpperSaturationLimit=2*pi  LowerSaturationLimit=-2*pi  ICPrevOutput=DiscIntNeverNeededParam  ICPrevScaledInput=DiscIntNeverNeededParam
  Mux{,1..3} (4 alike) : Mux  Inputs=2
  Rate Transition2 : RateTransition
  Visualization Gain1 : Gain  Gain=0.2
  Position Blade1 : Outport
  Position Blade 2 : Outport  Port=2
  Position Blade 3 : Outport  Port=3
  Position Blade 4 : Outport  Port=4
  wires:
  Bias3/1 -> Mux3/2
  Mux3/1 -> Position Blade 4/1
  Bias1/1 -> Mux1/2
  Bias2/1 -> Mux2/2
  Demux/2 -> Bias1/1
  Constant/1 -> Mux3/1, Mux2/1, Mux1/1, Mux/1
  Mux1/1 -> Position Blade 2/1
  Mux2/1 -> Position Blade 3/1
  Data Type Conversion/1 -> Visualization Gain1/1
  Discrete-Time Integrator/1 -> Rate Transition2/1
  Mux/1 -> Position Blade1/1
  Demux/3 -> Bias2/1
  Bias/1 -> Mux/2
  Prop_Rot_radPs/1 -> Data Type Conversion/1
  Demux/4 -> Bias3/1
  Rate Transition2/1 -> Demux/1
  Demux/1 -> Bias/1
  Visualization Gain1/1 -> Discrete-Time Integrator/1

== system MILSIM/Visualization/3D_Visualization/Matlab_3D/Visualization/Euler to VR/Axis Angle Vector ==
  e0 : Inport
  2 : Gain  Gain=2  SaturateOnIntegerOverflow=on  OutDataTypeStr=Inherit: Same as input  ParamDataTypeStr=Inherit: Same as input
  Constant : Constant  Value=1e-6
  Demux : Demux  Outputs=[1 3 ]
  Mux : Mux  Inputs=2
  Product : Product  Inputs=*/  SaturateOnIntegerOverflow=on  InputSameDT=on  OutDataTypeStr=Inherit: Same as first input
  Switch : Switch  Criteria=u2 ~= 0
  Trigonometric Function : Trigonometry
  Trigonometric Function2 : Trigonometry  Operator=acos
  e0_norm : Outport
  wires:
  Demux/1 -> Trigonometric Function2/1
  Demux/2 -> Product/1
  Mux/1 -> e0_norm/1
  Product/1 -> Mux/1
  2/1 -> Mux/2
  Trigonometric Function/1 -> Switch/1, Switch/2
  Trigonometric Function2/1 -> Trigonometric Function/1, 2/1
  e0/1 -> Demux/1
  Constant/1 -> Switch/3
  Switch/1 -> Product/2

== system MILSIM/Visualization/3D_Visualization/Matlab_3D/Visualization/Euler to VR/Quaternion Normalization ==
  e0 : Inport
  1/2 : Gain  Gain=1/2  SaturateOnIntegerOverflow=on  OutDataTypeStr=Inherit: Same as input  ParamDataTypeStr=Inherit: Same as input
  Demux : Demux  Outputs=[1 3]
  Mux : Mux  Inputs=2
  Product : Product  SaturateOnIntegerOverflow=on  InputSameDT=on  OutDataTypeStr=Inherit: Same as first input
  Trigonometric Function : Trigonometry
  Trigonometric Function1 : Trigonometry  Operator=cos
  e0_norm : Outport
  wires:
  Trigonometric Function1/1 -> Mux/1
  Demux/2 -> Product/2
  Demux/1 -> 1/2/1
  Mux/1 -> e0_norm/1
  Product/1 -> Mux/2
  Trigonometric Function/1 -> Product/1
  1/2/1 -> Trigonometric Function1/1, Trigonometric Function/1
  e0/1 -> Demux/1

== system MILSIM/Visualization/3D_Visualization/Matlab_3D/Visualization/Euler to VR/Quaternion Normalization1 ==
  e0 : Inport
  1/2 : Gain  Gain=1/2  SaturateOnIntegerOverflow=on  OutDataTypeStr=Inherit: Same as input  ParamDataTypeStr=Inherit: Same as input
  Demux : Demux  Outputs=[1 3]
  Mux : Mux  Inputs=2
  Product : Product  SaturateOnIntegerOverflow=on  InputSameDT=on  OutDataTypeStr=Inherit: Same as first input
  Trigonometric Function : Trigonometry
  Trigonometric Function1 : Trigonometry  Operator=cos
  e0_norm : Outport
  wires:
  e0/1 -> Demux/1
  1/2/1 -> Trigonometric Function/1, Trigonometric Function1/1
  Trigonometric Function/1 -> Product/1
  Product/1 -> Mux/2
  Mux/1 -> e0_norm/1
  Demux/1 -> 1/2/1
  Demux/2 -> Product/2
  Trigonometric Function1/1 -> Mux/1

== system MILSIM/Visualization/3D_Visualization/Matlab_3D/Visualization/Euler to VR/Quaternion Normalization2 ==
  e0 : Inport
  1/2 : Gain  Gain=1/2  SaturateOnIntegerOverflow=on  OutDataTypeStr=Inherit: Same as input  ParamDataTypeStr=Inherit: Same as input
  Demux : Demux  Outputs=[1 3]
  Mux : Mux  Inputs=2
  Product : Product  SaturateOnIntegerOverflow=on  InputSameDT=on  OutDataTypeStr=Inherit: Same as first input
  Trigonometric Function : Trigonometry
  Trigonometric Function1 : Trigonometry  Operator=cos
  e0_norm : Outport
  wires:
  Trigonometric Function1/1 -> Mux/1
  Demux/2 -> Product/2
  Demux/1 -> 1/2/1
  Mux/1 -> e0_norm/1
  Product/1 -> Mux/2
  Trigonometric Function/1 -> Product/1
  1/2/1 -> Trigonometric Function1/1, Trigonometric Function/1
  e0/1 -> Demux/1
